simulink model "model5_2_d"  (R2024b)
settings: Solver=FixedStepAuto  StartTime=0.0  StopTime=0.1  FixedStep=Ts  RelTol=1e-3
values from neighbouring files (symbols this model uses):
  Ts = 0.001    [domaci5_2_d.m]
  w = 2    [domaci5_2_d.m]    (also in domaci5_2_k.m = 20)
settings Model: Creator=neso  LastModifiedBy=neso

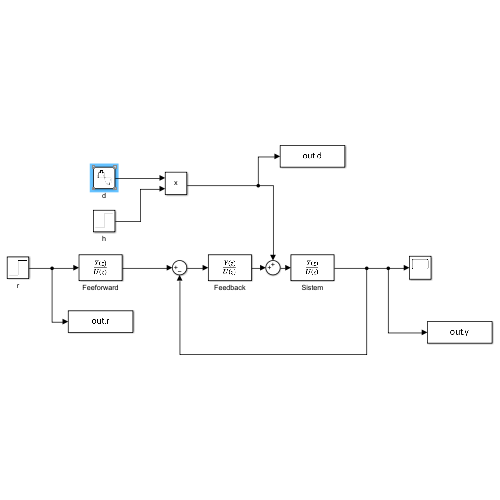
[thumbnail: Simulink's stored preview of the top-level diagram]
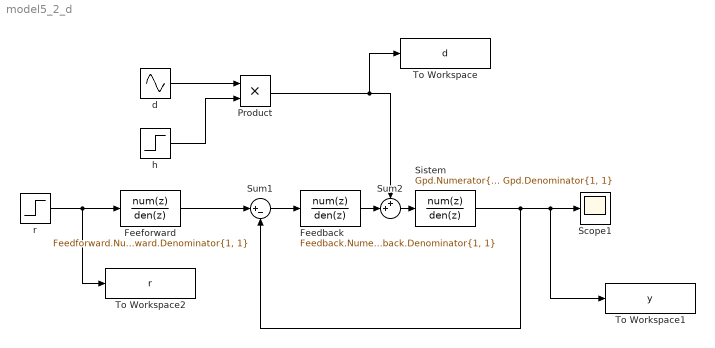
== system model5_2_d ==
  Feedback : DiscreteTransferFcn  Numerator=Feedback.Numerator{1, 1}  Denominator=Feedback.Denominator{1, 1}
  Feeforward : DiscreteTransferFcn  Numerator=Feedforward.Numerator{1, 1}  Denominator=Feedforward.Denominator{1, 1}
  Product : Product
  Scope1 : Scope
  Sistem : DiscreteTransferFcn  Numerator=Gpd.Numerator{1, 1}  Denominator=Gpd.Denominator{1, 1}
  Sum1 : Sum  Inputs=|+-
  Sum2 : Sum  Inputs=++|
  To Workspace : ToWorkspace  VariableName=d  SaveFormat=Timeseries  SampleTime=-1
  To Workspace1 : ToWorkspace  VariableName=y  SaveFormat=Timeseries  SampleTime=-1
  To Workspace2 : ToWorkspace  VariableName=r  SaveFormat=Timeseries  SampleTime=-1
  d : Sin  Amplitude=30  Frequency=w  SampleTime=Ts
  h : Step  Time=0.03  SampleTime=Ts
  r : Step  Time=0  After=5  SampleTime=Ts
  wires:
  r/1 -> To Workspace2/1, Feeforward/1
  Sistem/1 -> To Workspace1/1, Scope1/1, Sum1/2
  Sum1/1 -> Feedback/1
  Feeforward/1 -> Sum1/1
  Feedback/1 -> Sum2/2
  Sum2/1 -> Sistem/1
  d/1 -> Product/1
  h/1 -> Product/2
  Product/1 -> To Workspace/1, Sum2/1
